simulink model "Chua_4D"  (R2014b)
settings: Solver=ode45  StartTime=0.0  StopTime=10.0  RelTol=1e-3
values from neighbouring files (symbols this model uses):
  a = 0.95    [Run_Aizawa.m]    (also in Run_Arneodo.m = -5.5; Run_Chen.m = 33; Run_Chua.m = 15.6; Run_Chua_4D.m = 0.03)
  A = 30    [Run_Chua_4D.m]    (also in Run_FitzHugh_Nagumo.m = 0.8)
  B = 50    [Run_Chua_4D.m]
  c = -1    [Run_Arneodo.m]    (also in Run_Chen.m = 25; Run_Chua_4D.m = -1.2; Run_Dadras.m = 2; Run_HindmarshRose.m = 1)
  G = 0.32    [Run_Chua_4D.m]
  s = 3.5    [Run_Aizawa.m]    (also in Run_Chua_4D.m = 0.75; Run_Duffing.m = 0.2; Run_HindmarshRose.m = 4; Run_Lorenz.m = 10)
undefined symbols (not defined in the file or in its folder): param
settings Model: Creator=Arek  LastModifiedBy=Arek

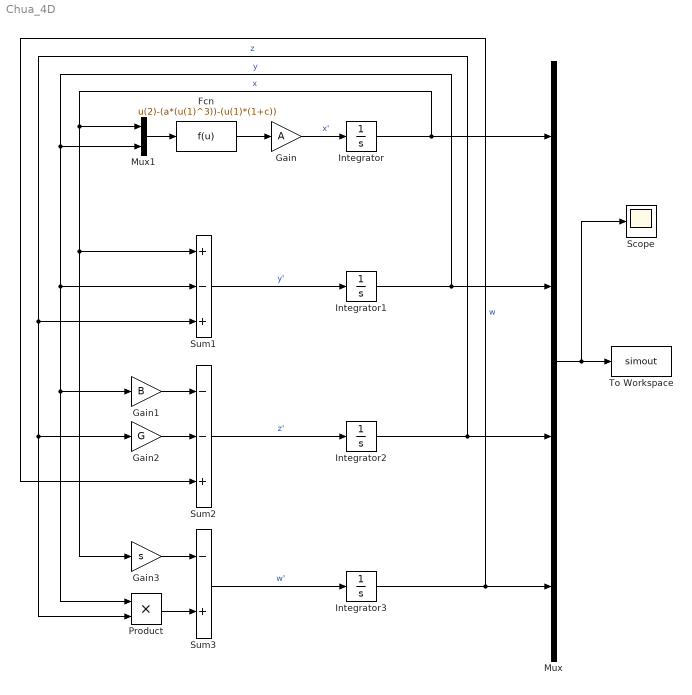
== system Chua_4D ==
  Fcn : Fcn  Expr=u(2)-(a*(u(1)^3))-(u(1)*(1+c))
  Gain : Gain  Gain=A
  Gain1 : Gain  Gain=B
  Gain2 : Gain  Gain=G
  Gain3 : Gain  Gain=s
  Integrator : Integrator  InitialCondition=param.ic(1)
  Integrator1 : Integrator  InitialCondition=param.ic(2)
  Integrator2 : Integrator  InitialCondition=param.ic(3)
  Integrator3 : Integrator  InitialCondition=param.ic(4)
  Mux : Mux
  Mux1 : Mux  Inputs=2
  Product : Product
  Scope : Scope
      settings: ShowLegends=on  TimeRange=0.05  YMin=-6  YMax=2
  Sum1 : Sum  Inputs=+-+
  Sum2 : Sum  Inputs=--+
  Sum3 : Sum  Inputs=-+
  To Workspace : ToWorkspace  VariableName=simout  SaveFormat=Timeseries  SampleTime=-1
  wires:
  Sum2/1 -> Integrator2/1  "z'"
  Sum1/1 -> Integrator1/1  "y'"
  Gain/1 -> Integrator/1  "x'"
  Integrator/1 -> Gain3/1, Sum1/1, Mux1/1, Mux/1  "x"
  Integrator1/1 -> Product/1, Gain1/1, Sum1/2, Mux1/2, Mux/2  "y"
  Integrator2/1 -> Product/2, Gain2/1, Sum1/3, Mux/3  "z"
  Mux/1 -> Scope/1, To Workspace/1
  Fcn/1 -> Gain/1
  Mux1/1 -> Fcn/1
  Integrator3/1 -> Sum2/3, Mux/4  "w"
  Gain1/1 -> Sum2/1
  Gain2/1 -> Sum2/2
  Product/1 -> Sum3/2
  Gain3/1 -> Sum3/1
  Sum3/1 -> Integrator3/1  "w'"
